simulink model "CarE_Model"  (R2019b)
settings: Solver=VariableStepAuto  StartTime=0.0  StopTime=inf  RelTol=1e-3
(part 4 of 5)

== matlab function CarE_Model/CarE_System/Emotion Module/Decay Module/Decay of Distress/MATLAB Function ==
  data: u input; y output; t input; ulast input
function y = fcn(u,t, ulast)
s = 100;
%local_t = t;

if(u == ulast)
    local_t = t-t;
else
    local_t = t-t+1;
end

if(u==0)
    y = 0;
else
    y = u -(local_t*100)/s;
end
end

== matlab function CarE_Model/CarE_System/Emotion Module/Decay Module/Decay of Fear/MATLAB Function ==
  data: u input; y output; t input; ulast input
function y = fcn(u,t, ulast)
s = 100;
%local_t = t;

if(u == ulast)
    local_t = t-t;
else
    local_t = t-t+1;
end

if(u==0)
    y = 0;
else
    y = u -(local_t*100)/s;
end
end

== matlab function CarE_Model/CarE_System/Mood Module/MATLAB Function1 ==
  data: previous_mood input; joy input; mood output; distress input; hope input; fear input; satisfaction input; fear_confirmed input; relief input; disappointment input; happy_for input; sorry_for input; gloating input; resentment input; pride input; shame input; admiration input; reproach input; gratitude input; anger input; gratification input; remorse input; liking input; disliking input; p output; n output; sort_positive output; index_positive output; sort_negative output; index_negative output; contribution output; index output; sum_of_contribution output; joy_driver input; distress_driver input; hope_driver input; fear_driver input; satisfaction_driver input; fear_confirmed_driver input; relief_driver input; disappointment_driver input; happy_for_driver input; sorry_for_driver input; gloating_driver input; resentment_driver input; pride_driver input; shame_driver input; admiration_driver input; reproach_driver input; gratitude_driver input; anger_driver input; gratification_driver input; remorse_driver input; liking_driver input; disliking_driver input
function [mood, p, n, sort_positive, index_positive, sort_negative, index_negative, contribution, index, sum_of_contribution] = mood_cal(previous_mood, joy, distress, hope, fear, satisfaction, fear_confirmed, relief, disappointment, happy_for, sorry_for, gloating, resentment, pride, shame, admiration, reproach, gratitude, anger, gratification, remorse, liking, disliking, joy_driver, distress_driver, hope_driver, fear_driver, satisfaction_driver, fear_confirmed_driver, relief_driver, disappointment_driver, happy_for_driver, sorry_for_driver, gloating_driver, resentment_driver, pride_driver, shame_driver, admiration_driver, reproach_driver, gratitude_driver, anger_driver, gratification_driver, remorse_driver, liking_driver, disliking_driver)
%psort = zeros(22,1);
positive_emo = 0;
negative_emo = 0;
individual_contribution_p = zeros(22,1);
individual_contribution_n = zeros(22,1);
positive_emo = positive_emo + abs(joy) + abs(hope) + abs(satisfaction) + abs(relief) + abs(happy_for) + abs(gloating) + abs(pride) + abs(admiration) + abs(gratitude) + abs(gratification) + abs(liking);
negative_emo = negative_emo + abs(distress) + abs(fear) + abs(fear_confirmed) + abs(disappointment) + abs(sorry_for) + abs(resentment) + abs(shame) + abs(reproach) + abs(anger) + abs(remorse) + abs(disliking);
p = positive_emo;
n = negative_emo;
if(negative_emo==0)
    negative_emo=1;
end
%% Finding the percentage contribution of each emotion in mood value
%assigning contributions to their respective arrays
%depending on if they are positive or negative
individual_contribution_p(1) = abs(joy)/positive_emo;
individual_contribution_n(2) = abs(distress)/negative_emo;
individual_contribution_p(3) = abs(hope)/positive_emo;
individual_contribution_n(4) = abs(fear)/negative_emo;
individual_contribution_p(5) = abs(satisfaction)/positive_emo;
individual_contribution_n(6) = abs(fear_confirmed)/negative_emo;
individual_contribution_p(7) = abs(relief)/positive_emo;
individual_contribution_n(8) = abs(disappointment)/negative_emo;
individual_contribution_p(9) = abs(happy_for)/positive_emo;
individual_contribution_n(10) = abs(sorry_for)/negative_emo;
individual_contribution_p(11) = abs(gloating)/positive_emo;
individual_contribution_n(12) = abs(resentment)/negative_emo;
individual_contribution_p(13) = abs(pride)/positive_emo;
individual_contribution_n(14) = abs(shame)/negative_emo;
individual_contribution_p(15) = abs(admiration)/positive_emo;
individual_contribution_n(16) = abs(reproach)/negative_emo;
individual_contribution_p(17) = abs(gratitude)/positive_emo;
individual_contribution_n(18) = abs(anger)/negative_emo;
individual_contribution_p(19) = abs(gratification)/positive_emo;
individual_contribution_n(20) = abs(remorse)/negative_emo;
individual_contribution_p(21) = abs(liking)/positive_emo;
individual_contribution_n(22) = abs(disliking)/negative_emo;

%First add the two arrays to combine the results in one array
combined_result = individual_contribution_p + individual_contribution_n;
%Sorting them in decreasing order
[contribution,index] = sort(combined_result, 'descend');
[sort_positive,index_positive] = sort(individual_contribution_p, 'descend');
[sort_negative,index_negative] = sort(individual_contribution_n, 'descend');
sum_of_contribution = sum(contribution);

%% calculating mood
if(negative_emo ~=0)
    mood = positive_emo/negative_emo;
else
    mood = previous_mood;
end

end

== matlab function CarE_Model/CarE_System/Emotion Module/Decay Module/Decay of Fear Confirmed/MATLAB Function ==
  data: u input; y output; t input; ulast input
function y = fcn(u,t, ulast)
s = 100;
%local_t = t;

if(u == ulast)
    local_t = t-t;
else
    local_t = t-t+1;
end

if(u==0)
    y = 0;
else
    y = u -(local_t*100)/s;
end
end

== matlab function CarE_Model/CarE_System/Emotion Module/Decay Module/Decay of Hope/MATLAB Function ==
  data: u input; y output; t input; ulast input
function y = fcn(u,t, ulast)
s = 100;
%local_t = t;

if(u == ulast)
    local_t = t-t;
else
    local_t = t-t+1;
end

if(u==0)
    y = 0;
else
    y = u -(local_t*100)/s;
end
end

== matlab function CarE_Model/CarE_System/Emotion Module/Decay Module/Decay of Disappointment/MATLAB Function ==
  data: u input; y output; t input; ulast input
function y = fcn(u,t, ulast)
s = 100;
%local_t = t;

if(u == ulast)
    local_t = t-t;
else
    local_t = t-t+1;
end

if(u==0)
    y = 0;
else
    y = u -(local_t*100)/s;
end
end

== matlab function CarE_Model/CarE_System/Emotion Module/Decay Module/Decay of Happy For/MATLAB Function ==
  data: u input; y output; t input; ulast input
function y = fcn(u,t, ulast)
s = 100;
%local_t = t;

if(u == ulast)
    local_t = t-t;
else
    local_t = t-t+1;
end

if(u==0)
    y = 0;
else
    y = u -(local_t*100)/s;
end
end

== matlab function CarE_Model/CarE_System/Emotion Module/Decay Module/Decay of Relief/MATLAB Function ==
  data: u input; y output; t input; ulast input
function y = fcn(u,t, ulast)
s = 100;
%local_t = t;

if(u == ulast)
    local_t = t-t;
else
    local_t = t-t+1;
end

if(u==0)
    y = 0;
else
    y = u -(local_t*100)/s;
end
end

== matlab function CarE_Model/CarE_System/Emotion Module/Decay Module/Decay of Gloating/MATLAB Function ==
  data: u input; y output; t input; ulast input
function y = fcn(u,t, ulast)
s = 100;
%local_t = t;

if(u == ulast)
    local_t = t-t;
else
    local_t = t-t+1;
end

if(u==0)
    y = 0;
else
    y = u -(local_t*100)/s;
end
end

== matlab function CarE_Model/CarE_System/Emotion Module/Decay Module/Decay of Resentment/MATLAB Function ==
  data: u input; y output; t input; ulast input
function y = fcn(u,t, ulast)
s = 100;
%local_t = t;

if(u == ulast)
    local_t = t-t;
else
    local_t = t-t+1;
end

if(u==0)
    y = 0;
else
    y = u -(local_t*100)/s;
end
end

== matlab function CarE_Model/CarE_System/Emotion Module/Decay Module/Decay of Pride/MATLAB Function ==
  data: u input; y output; t input; ulast input
function y = fcn(u,t, ulast)
s = 100;
%local_t = t;

if(u == ulast)
    local_t = t-t;
else
    local_t = t-t+1;
end

if(u==0)
    y = 0;
else
    y = u -(local_t*100)/s;
end
end

== matlab function CarE_Model/CarE_System/Emotion Module/Decay Module/Decay of Satisfaction/MATLAB Function ==
  data: u input; y output; t input; ulast input
function y = fcn(u,t, ulast)
s = 100;
%local_t = t;

if(u == ulast)
    local_t = t-t;
else
    local_t = t-t+1;
end

if(u==0)
    y = 0;
else
    y = u -(local_t*100)/s;
end
end

== matlab function CarE_Model/CarE_System/Emotion Module/Decay Module/Decay of Reproach/MATLAB Function ==
  data: u input; y output; t input; ulast input
function y = fcn(u,t, ulast)
s = 100;
%local_t = t;

if(u == ulast)
    local_t = t-t;
else
    local_t = t-t+1;
end

if(u==0)
    y = 0;
else
    y = u -(local_t*100)/s;
end
end

== matlab function CarE_Model/CarE_System/Emotion Module/Decay Module/Decay of Admiration/MATLAB Function ==
  data: u input; y output; t input; ulast input
function y = fcn(u,t, ulast)
s = 100;
%local_t = t;

if(u == ulast)
    local_t = t-t;
else
    local_t = t-t+1;
end

if(u==0)
    y = 0;
else
    y = u -(local_t*100)/s;
end
end

== matlab function CarE_Model/CarE_System/Emotion Module/Decay Module/Decay of Gratitude/MATLAB Function ==
  data: u input; y output; t input; ulast input
function y = fcn(u,t, ulast)
s = 100;
%local_t = t;

if(u == ulast)
    local_t = t-t;
else
    local_t = t-t+1;
end

if(u==0)
    y = 0;
else
    y = u -(local_t*100)/s;
end
end

== matlab function CarE_Model/CarE_System/Emotion Module/Decay Module/Decay of Anger/MATLAB Function ==
  data: u input; y output; t input; ulast input
function y = fcn(u,t, ulast)
s = 100;
%local_t = t;

if(u == ulast)
    local_t = t-t;
else
    local_t = t-t+1;
end

if(u==0)
    y = 0;
else
    y = u -(local_t*100)/s;
end
end

== matlab function CarE_Model/CarE_System/Emotion Module/Decay Module/Decay of Gratification/MATLAB Function ==
  data: u input; y output; t input; ulast input
function y = fcn(u,t, ulast)
s = 100;
%local_t = t;

if(u == ulast)
    local_t = t-t;
else
    local_t = t-t+1;
end

if(u==0)
    y = 0;
else
    y = u -(local_t*100)/s;
end
end

== matlab function CarE_Model/CarE_System/Emotion Module/Decay Module/Decay of Remorse/MATLAB Function ==
  data: u input; y output; t input; ulast input
function y = fcn(u,t, ulast)
s = 100;
%local_t = t;

if(u == ulast)
    local_t = t-t;
else
    local_t = t-t+1;
end

if(u==0)
    y = 0;
else
    y = u -(local_t*100)/s;
end
end

== matlab function CarE_Model/CarE_System/Emotion Module/Decay Module/Decay of Liking/MATLAB Function ==
  data: u input; y output; t input; ulast input
function y = fcn(u,t, ulast)
s = 100;
%local_t = t;

if(u == ulast)
    local_t = t-t;
else
    local_t = t-t+1;
end

if(u==0)
    y = 0;
else
    y = u -(local_t*100)/s;
end
end

== matlab function CarE_Model/CarE_System/Emotion Module/Decay Module/Decay of Disliking/MATLAB Function ==
  data: u input; y output; t input; ulast input
function y = fcn(u,t, ulast)
s = 100;
%local_t = t;

if(u == ulast)
    local_t = t-t;
else
    local_t = t-t+1;
end

if(u==0)
    y = 0;
else
    y = u -(local_t*100)/s;
end
end

== matlab function CarE_Model/CarE_System/Emotion Module/Decay Module/Decay of Shame/MATLAB Function ==
  data: u input; y output; t input; ulast input
function y = fcn(u,t, ulast)
s = 100;
%local_t = t;

if(u == ulast)
    local_t = t-t;
else
    local_t = t-t+1;
end

if(u==0)
    y = 0;
else
    y = u -(local_t*100)/s;
end
end

== matlab function CarE_Model/CarE_System/Emotion Module/Intensity Module/MATLAB Function to calculate individual emotion intensity ==
  data: goal_id input; agent_id input; event_id input; action_id input; LoS_0 input; LoF_0 input; fix input; joy output; distress output; hope output; fear output; satisfaction output; fear_confirmed output; relief output; disappointment output; happy_for output; sorry_for output; gloating output; resentment output; pride output; shame output; admiration output; reproach output; gratitude output; anger output; gratification output; remorse output; liking output; disliking output; sout output; fout output; sin input; fin input
function [joy, distress, hope, fear, satisfaction, fear_confirmed, relief, disappointment, happy_for, sorry_for, gloating, resentment, pride, shame, admiration, reproach, gratitude, anger, gratification, remorse, liking, disliking, sout, fout] = intensity_cal(goal_id, agent_id, event_id, action_id,LoS_0, LoF_0 , fix, sin, fin)
%% INITIALIZING
intensity.joy = 0;
intensity.distress = 0;
intensity.hope = 0;
intensity.fear = 0;
intensity.satisfaction = 0;
intensity.fear_confirmed = 0;
intensity.relief = 0;
intensity.disappointment = 0;
intensity.happy_for = 0;
intensity.sorry_for = 0;
intensity.gloating = 0;
intensity.resentment = 0;
intensity.pride = 0;
intensity.shame = 0;
intensity.admiration = 0;
intensity.reproach = 0;
intensity.gratitude = 0;
intensity.anger = 0;
intensity.gratification = 0;
intensity.remorse = 0;
intensity.liking = 0;
intensity.disliking = 0;

joy = 0;
distress = 0;
hope = 0;
fear = 0;
satisfaction = 0;
fear_confirmed = 0;
relief = 0;
disappointment = 0;
happy_for = 0;
sorry_for = 0;
gloating = 0;
resentment = 0;
pride = 0;
shame = 0;
admiration = 0;
reproach = 0;
gratitude = 0;
anger = 0;
gratification = 0;
remorse = 0;
liking = 0;
disliking = 0;

%% Defining LoS and LoF fix or as te stress factor
LoS=0.5;
LoF=0.5;
%fix=1;
coder.extrinsic('Cal_LoS')
[LoS,LoF]=Cal_LoS(goal_id,LoS_0, LoF_0 , fix);

%% DEFINING DATASET ARRAYS
%goal_set = [id number, name, hierarchy, desirability of success, desirability of not to fail, likelihood of success, likelihood of failure, related agent id];
goal_set = [
1, 100, 100, 100, 0.5, 0.5, 1; %"Stay under speed limit"
2, 95, 80, 70, LoS, LoF, 3;     %"Maintain proper distance with agents"
3, 85, 90, 75, LoS, LoF, 4;     %"Perform proper lane changes"
4, 100, 100, 100, 1, 0, 5;      %"Stop at red traffic light"
5, 95, 95, 90, 0.5, 0.5, 4;     %"Yield before turning"
6, 100, 100, 100, 1, 0, 6;     %"Avoid collision with pedestrians"
7, 100, 100, 100, LoS, LoF, 6;     %"Avoid collision with vehicles"
8, 85, 90, 75, LoS, LoF, 4];       % "Perform proper curve management"

%agent_set = [id number, name, type not_human|human, appealiness, related goal id];
agent_set = [1, 1, 100, -1;   %"ME (car itself)"
2, 1, 100, -1;              %"Driver"
3, 1, 90, 2;                %"Vehicle in front",
4, 1, 90, 2;                %"Vehicle in back" 
5, 0, 80, 4;                %"Traffic lights" 
6, 1, 100, 6;               %"Pedestrians" 
7, 0, 80, 6;                %"Animals" 
8, 0, 80, 6];               %"Buildings"

%event_set = [id number	name, change in goal LoS, change in goal LoF, related goal id];
event_set = [1, 1, -1, 1;   %"Staying under speed limit" 
2, -1, 1, 1;        %"Overspeeding detected" 
3, 1, -1, 2;        %"Proper distance maintained with agents" 
4, -1, 1, 2;        %"Improper distance maintained with agents"
5, 1, -1, 3;        %"Proper lane change performed" 
6, -0.75, 0.75, 3;  %"Improper lane change performed" 
7, 1, -1, 4;        %"Stopped at red light" 
8, -1, 1, 4;        %"Drove past red light" 
9, 1, -1, 5;        %"Yielded before turning" 
10, -0.5, 0.5, 5;   %"Turned without yielding" 
11, 1, -1, 6;       %"No collision detected" 
12, -1, 1, 6;      %"Collision detected" 
13, 1, -1, 3;        %"Proper curve handle performed" 
14, -0.75, 0.75, 3];  %"Improper curve handle performed" 

%action_set = [id number, name, praiseworthiness, related agent id, responsibility of the agent, related event id];
action_set = [1,  100, 2, 1, 1; %"I stayed in speed limit"
2, -90, 2, 1, 2;    %"I overspeeded" 
3, 100, 3, 1, 3;    %"I maintained proper distance with agents" 
4, -100, 3, 1, 4;    %"I maintained improper distance with agents" 
5, 80, 4, 1, 5;    %"I performed proper lane change" 
6, -80, 4, 1, 6;     %"I performed improper lane change" 
7, 100, 5, 1, 7;    %"I stopped at red light" 
8, -100, 5, 1, 8;    %"I drove past red light" 
9, 80, 4, 1, 9;   %"I yielded before turning" 
10, -80, 4, 1, 10;   %"I turned without yielding" 
11, 100, 6, 1, 11;   %"I detected no collision" 
12, -100, 6, 1, 12; %"I detected a collision" 
13, 90, 4, 1, 13;    %"I performed proper curve handle" 
14, -90, 4, 1, 14];     %"I performed improper curve handle" 

%% DEFINING STRUCTURES AND VARIABLES
%% ASSIGNING IMPORTED DATA TO VARIABLES
%GOAL
%if(goal_id ~= 0)
    goal.id = goal_set(goal_id,1);
    %goal.name = goal_set(goal_id,2);
    goal.hierarchy = goal_set(goal_id,2);
    goal.DoS = goal_set(goal_id,3);
    goal.DnF = goal_set(goal_id,4);
    goal.LoS = goal_set(goal_id,5);
    goal.LoF = goal_set(goal_id,6);
    goal.agent = goal_set(goal_id,7);
%end

%AGENT
%if(agent_id ~= 0)
    agent.id = agent_set(agent_id,1);
    %agent.name = agent_set(agent_id,2);
    agent.type = agent_set(agent_id,2);
    agent.appeal = agent_set(agent_id,3);
    agent.goal = agent_set(agent_id,4);
%end

%EVENT
%if(event_id ~= 0)
    event.id = event_set(event_id,1);
    %event.name = event_set(event_id,2);
    event.dLoS = event_set(event_id,2);
    event.dLoF = event_set(event_id,3);
    event.goal = event_set(event_id,4);
%end

%ACTION
%if(action_id ~= 0)
    action.id = action_set(action_id,1);
    %action.name = action_set(action_id,2);
    action.praise = action_set(action_id,2);
    action.agent = action_set(action_id,3);
    action.resp = action_set(action_id,4);
    action.event = action_set(action_id,5);
%end
sout = goal.LoS;
fout = goal.LoF;
last.LoS = sin;
last.LoF = fin;
% last.LoS = 0.5;
% last.LoF = 0.5;
no_emotion = 0;


%% FINDING EMOTION INTENSITY VALUES

% HOPE OR FEAR
if(goal.LoS > goal.LoF)
    intensity.hope = goal.LoS * goal.DoS;
    hope = intensity.hope;
    intensity.fear = no_emotion;
    fear = intensity.fear;
else
    intensity.fear = goal.LoF * goal.DnF;
    fear = intensity.fear;
    intensity.hope = no_emotion;
    hope = intensity.hope;
end

% LIKE OR DISLIKE
if(agent.appeal > 0)
    intensity.liking = agent.appeal;
    liking = intensity.liking;
    intensity.disliking = no_emotion;
    disliking = intensity.disliking;
else
    intensity.disliking = agent.appeal;
    disliking = intensity.disliking;
    intensity.liking = no_emotion;
    liking = intensity.liking;
end

% PRIDE OR SHAME - ADMIRATION OR REPROACH
if(agent.id==1)
    intensity.admiration = no_emotion;
    admiration = intensity.admiration;
    intensity.reproach = no_emotion;
    reproach = intensity.reproach;
    if(action.praise>0)
        intensity.pride = action.praise;
        pride = intensity.pride;
        intensity.shame = no_emotion;
        shame = intensity.shame;
    else
        intensity.shame = action.praise;
        shame = intensity.shame;
        intensity.pride = no_emotion;
        pride = intensity.pride;
    end
elseif(agent.id~=0)
    intensity.pride = no_emotion;
    pride = intensity.pride;
    intensity.shame = no_emotion;
    shame = intensity.shame;
    if(action.praise>0)
        intensity.admiration = action.praise;
        admiration = intensity.admiration;
        intensity.reproach = no_emotion;
        reproach = intensity.reproach;
    else
        intensity.reproach = action.praise;
        reproach = intensity.reproach;
        intensity.admiration = no_emotion;
        admiration = intensity.admiration;
    end
end

% GRATIFICATION OR GRATITUDE - REMORSE OR ANGER
if(event.dLoS > 0 && event.dLoF <= 0)
    intensity.remorse = no_emotion;
    remorse = intensity.remorse;
    intensity.anger = no_emotion;
    anger = intensity.anger;
	if(agent.id == 1)
		intensity.gratification = goal.DoS * action.resp;
    	gratification = intensity.gratification;
		intensity.gratitude = no_emotion;
    	gratitude = intensity.gratitude;
	else
		intensity.gratitude = goal.DoS * action.resp;
    	gratitude = intensity.gratitude;
		intensity.gratification = no_emotion;
   		gratification = intensity.gratification;
	end
else
    intensity.gratification = no_emotion;
   	gratification = intensity.gratification;
    intensity.gratitude = no_emotion;
    gratitude = intensity.gratitude;
    if(event.dLoF > 0 && event.dLoS <= 0)
        if(agent.id == 1)
            intensity.remorse = goal.DnF * action.resp;
            remorse = intensity.remorse;
            intensity.anger = no_emotion;
            anger = intensity.anger;
        else
            intensity.anger = goal.DnF * action.resp;
            anger = intensity.anger;
            intensity.remorse = no_emotion;
            remorse = intensity.remorse;
        end
    else
        intensity.gratification = no_emotion;
        gratification = intensity.gratification;
        intensity.gratitude = no_emotion;
        gratitude = intensity.gratitude;        
        intensity.remorse = no_emotion;
        remorse = intensity.remorse;
        intensity.anger = no_emotion;
        anger = intensity.anger;

    end
end

%JOY OR DISTRESS - HAPPY-FOR OR RESENTMENT - SORRY-FOR OR GLOATING
if(agent.id == 1)
    intensity.happy_for = no_emotion;
    happy_for = intensity.happy_for;
    intensity.resentment = no_emotion;
    resentment = intensity.resentment;
    intensity.sorry_for = no_emotion;
    sorry_for = intensity.sorry_for;
    intensity.gloating = no_emotion;
    gloating = intensity.gloating;
    if(event.dLoS>0 && event.dLoF<=0)
        intensity.joy = event.dLoS * goal.DoS;
        joy = intensity.joy;
        intensity.distress = no_emotion;
        distress = intensity.distress;
    else
        intensity.joy = no_emotion;
        joy = intensity.joy;
        if(event.dLoF>0 && event.dLoS<=0)
            intensity.distress = event.dLoF * goal.DnF;
            distress = intensity.distress;
        else
            intensity.joy = no_emotion;
            joy = intensity.joy;
            intensity.distress = no_emotion;
            distress = intensity.distress;
        end
    end
elseif(agent.id~=1)
    intensity.joy = no_emotion;
    joy = intensity.joy;
    intensity.distress = no_emotion;
    distress = intensity.distress;
    if(event.dLoS>0 && event.dLoF<=0)
        intensity.sorry_for = no_emotion;
        sorry_for = intensity.sorry_for;
        intensity.gloating = no_emotion;
        gloating = intensity.gloating;
        if(agent.appeal>0)
            intensity.happy_for = abs(agent.appeal) * event.dLoS * goal.DoS;
            happy_for = intensity.happy_for;
            intensity.resentment = no_emotion;
            resentment = intensity.resentment;
        else
            intensity.resentment = abs(agent.appeal) * event.dLoS * goal.DoS;
            resentment = intensity.resentment;
            intensity.happy_for = no_emotion;
            happy_for = intensity.happy_for;
        end
    else
        intensity.happy_for = no_emotion;
        happy_for = intensity.happy_for;
        intensity.resentment = no_emotion;
        resentment = intensity.resentment;
        if(event.dLoF>0 && event.dLoS<=0)
            if(agent.appeal>0)
                intensity.sorry_for = abs(agent.appeal) * event.dLoF * goal.DnF;
                sorry_for = intensity.sorry_for;
                intensity.gloating = no_emotion;
                gloating = intensity.gloating;
            else
                intensity.gloating = abs(agent.appeal) * event.dLoF * goal.DnF;
                gloating = intensity.gloating;
                intensity.sorry_for = no_emotion;
                sorry_for = intensity.sorry_for;
            end
        else
            intensity.happy_for = no_emotion;
            happy_for = intensity.happy_for;
            intensity.resentment = no_emotion;
            resentment = intensity.resentment;
            intensity.sorry_for = no_emotion;
            sorry_for = intensity.sorry_for;
            intensity.gloating = no_emotion;
            gloating = intensity.gloating;
        end
    end
end

%SATISFACTION OR DISAPPOINTMENT - FEAR-CONFIRMED OR RELIEF
if(last.LoS > last.LoF)
    intensity.fear_confirmed = no_emotion;
    fear_confirmed = intensity.fear_confirmed;
    intensity.relief = no_emotion;
    relief = intensity.relief;
    if(goal.LoS == 1)
        intensity.satisfaction = last.LoS * goal.DoS;
        satisfaction = intensity.satisfaction;
        intensity.disappointment = no_emotion;
        disappointment = intensity.disappointment;
    else
        intensity.satisfaction = no_emotion;
        satisfaction = intensity.satisfaction;
        if(goal.LoF == 1)
            intensity.disappointment = last.LoS * goal.DoS;
            disappointment = intensity.disappointment;
        else
            intensity.satisfaction = no_emotion;
            satisfaction = intensity.satisfaction;
            intensity.disappointment = no_emotion;
            disappointment = intensity.disappointment;
        end
    end
else
    intensity.satisfaction = no_emotion;
    satisfaction = intensity.satisfaction;
    intensity.disappointment = no_emotion;
    disappointment = intensity.disappointment;
    if(goal.LoS == 1)
        intensity.relief = last.LoF * goal.DnF;
        relief = intensity.relief;
        intensity.fear_confirmed = no_emotion;
        fear_confirmed = intensity.fear_confirmed;
    else
        intensity.relief = no_emotion;
        relief = intensity.relief;
        if(goal.LoF == 1)
            intensity.fear_confirmed = last.LoF * goal.DnF;
            fear_confirmed = intensity.fear_confirmed;
        else
            intensity.relief = no_emotion;
            relief = intensity.relief;
            intensity.fear_confirmed = no_emotion;
            fear_confirmed = intensity.fear_confirmed;
        end
    end
end

%% NORMALIZED VALUES
joy = inter(joy, 0, 100);
distress = inter(distress, 0, 100);
hope = inter(hope, 0, 100);
fear = inter(fear, 0, 100);
satisfaction = inter(satisfaction, 0, 100);
fear_confirmed = inter(fear_confirmed, 0, 100);
relief = inter(relief, 0, 100);
disappointment = inter(disappointment, 0, 100);
happy_for = inter(happy_for, 0, 10000);     %these values were too big and had to be interpolated to fit in 0-100 range
sorry_for = inter(sorry_for, 0, 10000);
gloating = inter(gloating, 0, 10000);
resentment = inter(resentment, 0, 10000);
pride = inter(pride, 0, 100);
shame = inter(shame, 0, 100);
admiration = inter(admiration, 0, 100);
reproach = inter(reproach, 0, 100);
gratitude = inter(gratitude, 0, 100);
anger = inter(anger, 0, 100);
gratification = inter(gratification, 0, 100);
remorse = inter(remorse, 0, 100);
liking = inter(liking, 0, 100);
disliking = inter(disliking, 0, 100);

%% NORMALIZING VALUES
% INTERPOLATION FUNCTION NEW
function interpolated = inter(a_val, low_th, high_th)
    if(a_val<0)
        y1 = -100;
        %y2 = 0;
        y3 = 0;
        x1 = -high_th;
        x2 = a_val;
        x3 = -low_th;
    else
        y1 = 100;
        %y2 = 0;
        y3 = 0;
        x1 = high_th;
        x2 = a_val;
        x3 = low_th;
    end
    %calculate the interpolated value    
    y2 = (((x2-x1)*(y3-y1))/(x3-x1))+y1;
    interpolated = y2;
end

end

== matlab function CarE_Model/CarE_System/Emotion Module/Decay Module/Decay of Joy/MATLAB Function1 ==
  data: u input; y output; t input; ulast input
function y = fcn(u,t, ulast)
% u - emotion intensity value
% ulast - emotion intensity in last instance of time
% t - timer value (age of emotion)
% s - max decay time
% y - decayed emotion intensity
s = 100;

if(u == ulast)
    local_t = t-t;
else
    local_t = t-t+1;
end

if(u==0)
    y = 0;
else
    y = u -(local_t*100)/s;
end
end

== matlab function CarE_Model/CarE_System/Emotion Module/Decay Module/Decay of Sorry For/MATLAB Function ==
  data: u input; y output; t input; ulast input
function y = fcn(u,t, ulast)
s = 100;
%local_t = t;

if(u == ulast)
    local_t = t-t;
else
    local_t = t-t+1;
end

if(u==0)
    y = 0;
else
    y = u -(local_t*100)/s;
end
end

== matlab function CarE_Model/CarE_System/Input_module_2.0/MATLAB Function ==
  data: distance input; brakes_st output; serv_brake_PE_st output; second_brake_st output; parking_brake_st output; axle_st output; warn_lamp_st output; door_st output; fog_lamp_st output; headlamp_st output; reverse_lamp_st output; belts_st output; airbag_st output; seat_st output; steering_st output; wheel_alignment_st output; EPS_st output; Steering_wheel_st output; stop_lamp_st output; suspension_st output; Telltales_st output; wheel_hub_st output; wheel_st output; tyre_st output; cabine_st output; chassis_st output
function [brakes_st,serv_brake_PE_st,second_brake_st,parking_brake_st,axle_st,warn_lamp_st,door_st,fog_lamp_st,headlamp_st,reverse_lamp_st,belts_st,airbag_st,seat_st,steering_st,wheel_alignment_st,EPS_st,Steering_wheel_st,stop_lamp_st,suspension_st,Telltales_st,wheel_hub_st,wheel_st,tyre_st,cabine_st,chassis_st]= state_VH(distance)
coder.extrinsic('VH_fun_state')
brakes_st=1;
serv_brake_PE_st=1;
second_brake_st=1;
parking_brake_st=1;
axle_st=1;
warn_lamp_st=1;
door_st=1;
fog_lamp_st=1;
headlamp_st=1;
reverse_lamp_st=1;
belts_st=1;
airbag_st=1;
seat_st=1;
steering_st=1;
wheel_alignment_st=1;
EPS_st=1;
Steering_wheel_st=1;
stop_lamp_st=1;
suspension_st=1;
Telltales_st=1;
wheel_hub_st=1;
wheel_st=1;
tyre_st=1;
cabine_st=1;
chassis_st=1;

[brakes_st,serv_brake_PE_st,second_brake_st,parking_brake_st,axle_st,warn_lamp_st,door_st,fog_lamp_st,headlamp_st,reverse_lamp_st,belts_st,airbag_st,seat_st,steering_st,wheel_alignment_st,EPS_st,Steering_wheel_st,stop_lamp_st,suspension_st,Telltales_st,wheel_hub_st,wheel_st,tyre_st,cabine_st,chassis_st]= VH_fun_state(distance);
end

== matlab function CarE_Model/CarE_System/Input_module_2.0/MATLAB Function1 ==
  data: avg_gap input; gap_st output; gap input
function gap_st  = gap_st_fun(avg_gap,gap)
coder.extrinsic('gap_st_comp');
gap_st=1;
gap_st  = gap_st_comp(avg_gap,gap);

end

== matlab function CarE_Model/CarE_System/Input_module_2.0/MATLAB Function2 ==
  data: obt_recog input; ob_recog_st output
function ob_recog_st = ob_recog_st_fun(obt_recog)
    coder.extrinsic('ob_recog_st_comp');
    ob_recog_st=1;
       ob_recog_st = ob_recog_st_comp(obt_recog);
end

== matlab function CarE_Model/CarE_System/Input_module_2.0/MATLAB Function3 ==
  data: acc_road_today input; prob_acc_road_st output; mean_acc input; SD_acc_road input
function prob_acc_road_st = prob_acc_road_st_funtion(acc_road_today,mean_acc,SD_acc_road)
    
    coder.extrinsic('prob_acc_road_st_fun');
      %coder.extrinsic('normcdf');
      prob_acc_road_st=1;
    prob_acc_road_st = prob_acc_road_st_fun(acc_road_today,mean_acc,SD_acc_road);
end

== matlab function CarE_Model/CarE_System/Health_Module_2.0/MATLAB Function ==
  data: driver_age_st input; HealthFactor output; driver_alcohol_st input; driver_alertness_st input; driver_vision_st input; driver_work_load_st input; driver_emotion_st input; driver_attitude_st input; maintenance_periodicity_st input; gap_st input; speeding_freq_st input; vehicle_mass_st input; brakes_st input; serv_brake_PE_st input; second_brake_st input; parking_brake_st input; axle_st input; warn_lamp_st input; door_st input; fog_lamp_st input; headlamp_st input; reverse_lamp_st input; belts_st input; airbag_st input; seat_st input; steering_st input; wheel_alignment_st input; EPS_st input; Steering_wheel_st input; stop_lamp_st input; suspension_st input; Telltales_st input; wheel_hub_st input; wheel_st input; tyre_st input; cabine_st input; chassis_st input; noise_st input; obt_recog_st input; v2v_st input; v2i_st input; friendly_HM_interaction_st input; software_freq_st input; biddata_connection_st input; digital_user_interface_st input; cooperative_driving_st input; road_surface_st input; road_condition_st input; prob_acc_road_st input; prob_contruction_st input; cab_temperature_st input; cab_humidity_st input; driving_env_condition_st input; weather_st input; time_of_day_st input; check_if_hit input; check_collision input
function HealthFactor = HeatlFactor_fun(driver_age_st,driver_alcohol_st,driver_alertness_st,driver_vision_st,driver_work_load_st,driver_emotion_st,driver_attitude_st,maintenance_periodicity_st,gap_st,speeding_freq_st,vehicle_mass_st,brakes_st,serv_brake_PE_st,second_brake_st,parking_brake_st,axle_st,warn_lamp_st,door_st,fog_lamp_st,headlamp_st,reverse_lamp_st,belts_st,airbag_st,seat_st,steering_st,wheel_alignment_st,EPS_st,Steering_wheel_st,stop_lamp_st,suspension_st,Telltales_st,wheel_hub_st,wheel_st,tyre_st,cabine_st,chassis_st,noise_st,obt_recog_st,v2v_st,v2i_st,friendly_HM_interaction_st,software_freq_st,biddata_connection_st,digital_user_interface_st,cooperative_driving_st,road_surface_st,road_condition_st,prob_acc_road_st,prob_contruction_st,cab_temperature_st,cab_humidity_st,driving_env_condition_st,weather_st,time_of_day_st,check_if_hit,check_collision)
HealthFactor=1;
coder.extrinsic('HealthFactor_fn')

HealthFactor = HealthFactor_fn(driver_age_st,driver_alcohol_st,driver_alertness_st,driver_vision_st,driver_work_load_st,driver_emotion_st,driver_attitude_st,maintenance_periodicity_st,gap_st,speeding_freq_st,vehicle_mass_st,brakes_st,serv_brake_PE_st,second_brake_st,parking_brake_st,axle_st,warn_lamp_st,door_st,fog_lamp_st,headlamp_st,reverse_lamp_st,belts_st,airbag_st,seat_st,steering_st,wheel_alignment_st,EPS_st,Steering_wheel_st,stop_lamp_st,suspension_st,Telltales_st,wheel_hub_st,wheel_st,tyre_st,cabine_st,chassis_st,noise_st,obt_recog_st,v2v_st,v2i_st,friendly_HM_interaction_st,software_freq_st,biddata_connection_st,digital_user_interface_st,cooperative_driving_st,road_surface_st,road_condition_st,prob_acc_road_st,prob_contruction_st,cab_temperature_st,cab_humidity_st,driving_env_condition_st,weather_st,time_of_day_st,check_if_hit,check_collision);


end

== matlab function CarE_Model/CarE_System/Event_detect_module/MATLAB Function ==
  data: egocar_x input; event_id output; egocar_z input; egocar_rot input; olanecar_presence input; leadcar_presence input; turn_trigger input
function event_id = Event_recognition(egocar_x,egocar_z,egocar_rot,olanecar_presence, leadcar_presence,turn_trigger)

%straight line lane change
%ode_wide=8; %unity units
event_id=1;
coder.extrinsic('Event_identification');
event_id = Event_identification(egocar_x,egocar_z,egocar_rot,olanecar_presence, leadcar_presence,turn_trigger);

%{
w_ego_car=1.58; %unity units
lanechange_trigger=0;
    if egocar_rot>=45 && egocar_rot<=135      
        lane_position=816;%z coordinate
        egocar_l=egocar_z-w_ego_car/2;
        egocar_r=egocar_z+w_ego_car/2; 
        direction=1;
    elseif egocar_rot>=225 && egocar_rot<=315
        lane_position=962; %z coordianates
        egocar_l=egocar_z+w_ego_car/2;
        egocar_r=egocar_z-w_ego_car/2;
        direction=-1;
    elseif egocar_rot>135 && egocar_rot<225
        lane_position=954;%xcoordinates
        egocar_l=egocar_x-w_ego_car/2;
        egocar_r=egocar_x+w_ego_car/2;
        direction=1;
    elseif egocar_rot>315 && egocar_rot<=360 || egocar_rot>=0 && egocar_rot<45
        lane_position=752.5;%xcoordinates
         egocar_l=egocar_x+w_ego_car/2;
        egocar_r=egocar_x-w_ego_car/2;
        direction=-1;
    end
    
     if egocar_l>lane_position && direction==1 || egocar_r<lane_position && direction==1
           lanechange_trigger=0;
     elseif egocar_l<lane_position && direction==-1 || egocar_r>lane_position && direction==-1
           lanechange_trigger=0;
     end
      
     if  direction ==1 && egocar_l<=lane_position && egocar_r>=lane_position
         lanechange_trigger=1;
     elseif direction ==-1 && egocar_l>=lane_position && egocar_r<=lane_position
         lanechange_trigger=1;
     end


    if olanecar_presence==1 && leadcar_presence==1 && lanechange_trigger==1 || olanecar_presence==0 && leadcar_presence==1 && lanechange_trigger==1
            event_id=5;
    elseif olanecar_presence==0 && leadcar_presence==1 && lanechange_trigger==0
            event_id=4;
    elseif lanechange_trigger==1 && olanecar_presence==0 && leadcar_presence==0 && turn_trigger==0
            event_id=3;
    elseif turn_trigger==1 && olanecar_presence==0 && leadcar_presence==0
            event_id=2;
    else
        event_id=1;
    end
    %}
end

== matlab function CarE_Model/CarE_System/Personality_module/MATLAB Function ==
  data: speed input; x output; max_speed input; max_x output
function [x,max_x] = Gain_fun(speed,max_speed)

    x=speed;
    max_x=max_speed;
end

== matlab function CarE_Model/CarE_System/Personality_module/MATLAB Function1 ==
  data: x input; U output; r input; max_x input
function U = Utility_fun(x,r,max_x)

    if x==0
        U_temp=0;
    else
        if r>=1
            r=0.999;
        end
        U_temp=((x)^(1-r))/(1-r);
    end
        max_U=((max_x)^(1-r))/(1-r);
        U=U_temp/max_U;

end

== matlab function CarE_Model/CarE_System/Stress_module/MATLAB Function ==
  data: distance input; SF_VH output
function SF_VH  = SF_VH_fun(distance)
    SF_VH=0;
    coder.extrinsic('SfactorVH_fun')
    SF_VH=SfactorVH_fun(distance);

end

== matlab function CarE_Model/CarE_System/Stress_module/MATLAB Function1 ==
  data: Mean_acc_road input; SF_Env output; SD_acc_road input; acc_road_today input; road_surface_st input; road_cond_st input; weather_st input; time_day_st input; egocar_speed input; avgspeed_data input
function SF_Env = SF_Env_fun(Mean_acc_road,SD_acc_road,acc_road_today,road_surface_st,road_cond_st,weather_st,time_day_st,egocar_speed,avgspeed_data)
    SF_Env=0;
    coder.extrinsic('SfactorEnv_fun')
    SF_Env=SfactorEnv_fun(Mean_acc_road,SD_acc_road,acc_road_today,road_surface_st,road_cond_st,weather_st,time_day_st,egocar_speed,avgspeed_data);
end

== matlab function CarE_Model/CarE_System/Stress_module/MATLAB Function2 ==
  data: Prob_obj_detec input; SF_VC output; v2v_st input; v2i_st input; bd_conect_st input; coop_auto_st input
function SF_VC  = SF_VC_fun(Prob_obj_detec,v2v_st,v2i_st,bd_conect_st,coop_auto_st)
    SF_VC=0;
    coder.extrinsic('SfactorVC_fun')
    SF_VC=SfactorVC_fun(Prob_obj_detec,v2v_st,v2i_st,bd_conect_st,coop_auto_st);
end

== matlab function CarE_Model/CarE_System/Stress_module/MATLAB Function3 ==
  data: speed_ecar input; SF_driving output; a_vehicle input; event_id input; gravity input; avg_speed input; rate_acc input; rate_desacc input; crit_gap input; pos_ecar_x input; pos_ecar_z input; rot_ecar input; pos_lead_car_x input; pos_lead_car_z input; speed_lead_car input; olanecar_presence input; pos_olane_car_x input; pos_olane_car_z input; rot_olane_car input; speed_olane_car input; gap output; check_if_hit input; collisiondetection input
function  [SF_driving,gap]= SF_driving_fun(speed_ecar,a_vehicle,event_id,gravity,avg_speed,rate_acc,rate_desacc,crit_gap,pos_ecar_x,pos_ecar_z,rot_ecar,pos_lead_car_x,pos_lead_car_z,speed_lead_car,olanecar_presence,pos_olane_car_x,pos_olane_car_z,rot_olane_car,speed_olane_car,check_if_hit,collisiondetection)
%%%%%%%%%%%%%%%%%%%%%%%%%%%%%%%%%%%%%
%{
possible events:
- driving alone
    -straingt line. event_id=1
    -curve. event_id=2
    -lane change. event_id=3 
- driving with another car
    -following another car. event_id=4
    -overtake. event_id=5
%}
%%%%%%%%%%%%%%%%%%%%%%%%%%%%%%%%%%%%%
    SF_driving=0;
    gap=1;
    coder.extrinsic('SF_driving_fun') 
    [SF_driving,gap]= SF_driving_fun(speed_ecar,a_vehicle,event_id,gravity,avg_speed,rate_acc,rate_desacc,crit_gap,pos_ecar_x,pos_ecar_z,rot_ecar,pos_lead_car_x,pos_lead_car_z,speed_lead_car,olanecar_presence,pos_olane_car_x,pos_olane_car_z,rot_olane_car,speed_olane_car,check_if_hit,collisiondetection);
end

== matlab function CarE_Model/CarE_System/Stress_module/MATLAB Function4 ==
  data: SF_VH input; SF output; SF_Env input; SF_VC input; SF_driving input
function SF = SF_cal(SF_VH,SF_Env,SF_VC,SF_driving)
    P1=SF_VH+SF_Env-SF_VH*SF_Env;
    P2=P1+SF_VC-P1*SF_VC;
    %SF=SF_VC+SF_Env+SF_VH+SF_driving-(SF_VC*SF_Env+SF_VC*SF_VH+SF_VH*SF_Env+SF_driving*SF_VC+SF_driving*SF_Env+SF_driving*SF_VH)+SF_VH*SF_Env*SF_VC*SF_driving;
    SF=P2+SF_driving-P2*SF_driving;
end

== matlab function CarE_Model/CarE_System/Emotion_Intensity_Input_Module/MATLAB Function ==
  data: event_0 input; goal_id output; event_detected input; sf_total input; check_hit input; check_trigger input; check_collision input; gap_st input; egocar_speed input; agent_id output; event_id output; action_id output; LoS output; LoF output; max_speed input
function [goal_id,agent_id,event_id,action_id,LoS,LoF] = Intensity_input(event_0,event_detected,sf_total,  check_hit,check_trigger,check_collision,gap_st,egocar_speed,max_speed)
  
  goal_id=1;
  agent_id=1;
  event_id=1;
  action_id=1;
  LoS=0.5;
  LoF=0.5;
  coder.extrinsic('e_intensity_detect');
[goal_id,agent_id,event_id,action_id,LoS,LoF] = e_intensity_detect(event_0,event_detected,sf_total,check_hit,check_trigger,check_collision,gap_st,egocar_speed,max_speed);
        
     



    end

== matlab function CarE_Model/CarE_System/Input_module_2.0/MATLAB Function4 ==
  data: driver_age_st input; driver_alcohol_st input; driver_alertness_st input; driver_vision_st input; driver_work_load_st input; driver_emotion_st input; driver_attitude_st input; maintenance_periodicity_st input; gap_st input; speeding_freq_st input; vehicle_mass_st input; brakes_st input; serv_brake_PE_st input; second_brake_st input; parking_brake_st input; axle_st input; warn_lamp_st input; door_st input; fog_lamp_st input; headlamp_st input; reverse_lamp_st input; belts_st input; airbag_st input; seat_st input; steering_st input; wheel_alignment_st input; EPS_st input; Steering_wheel_st input; stop_lamp_st input; suspension_st input; Telltales_st input; wheel_hub_st input; wheel_st input; tyre_st input; cabine_st input; chassis_st input; noise_st input; obt_recog_st input; v2v_st input; v2i_st input; friendly_HM_interaction_st input; software_freq_st input; biddata_connection_st input; digital_user_interface_st input; cooperative_driving_st input; road_surface_st input; road_condition_st input; prob_acc_road_st input; prob_contruction_st input; cab_temperature_st input; cab_humidity_st input; driving_env_condition_st input; weather_st input; time_of_day_st input; driver_age_st output; check_if_hit input; check_collision input; driver_alcohol_st output; driver_alertness_st output; driver_vision_st output; driver_work_load_st output; driver_emotion_st output; driver_attitude_st output; maintenance_periodicity_st output; gap_st output; speeding_freq_st output; vehicle_mass_st output; brakes_st output; serv_brake_PE_st output; second_brake_st output; parking_brake_st output; axle_st output; warn_lamp_st output; door_st output; fog_lamp_st output; headlamp_st output; reverse_lamp_st output; belts_st output; airbag_st output; seat_st output; steering_st output; wheel_alignment_st output; EPS_st output; Steering_wheel_st output; stop_lamp_st output; suspension_st output; Telltales_st output; wheel_hub_st output; wheel_st output; tyre_st output; cabine_st output; chassis_st output; noise_st output; obt_recog_st output; v2v_st output; v2i_st output; friendly_HM_interaction_st output; software_freq_st output; biddata_connection_st output; digital_user_interface_st output; cooperative_driving_st output; road_surface_st output; road_condition_st output; prob_acc_road_st output; prob_contruction_st output; cab_temperature_st output; cab_humidity_st output; driving_env_condition_st output; weather_st output; time_of_day_st output
function [driver_age_st,driver_alcohol_st,driver_alertness_st,driver_vision_st,driver_work_load_st,driver_emotion_st,driver_attitude_st,maintenance_periodicity_st,gap_st,speeding_freq_st,vehicle_mass_st,brakes_st,serv_brake_PE_st,second_brake_st,parking_brake_st,axle_st,warn_lamp_st,door_st,fog_lamp_st,headlamp_st,reverse_lamp_st,belts_st,airbag_st,seat_st,steering_st,wheel_alignment_st,EPS_st,Steering_wheel_st,stop_lamp_st,suspension_st,Telltales_st,wheel_hub_st,wheel_st,tyre_st,cabine_st,chassis_st,noise_st,obt_recog_st,v2v_st,v2i_st,friendly_HM_interaction_st,software_freq_st,biddata_connection_st,digital_user_interface_st,cooperative_driving_st,road_surface_st,road_condition_st,prob_acc_road_st,prob_contruction_st,cab_temperature_st,cab_humidity_st,driving_env_condition_st,weather_st,time_of_day_st] = input_collision_affect(driver_age_st,driver_alcohol_st,driver_alertness_st,driver_vision_st,driver_work_load_st,driver_emotion_st,driver_attitude_st,maintenance_periodicity_st,gap_st,speeding_freq_st,vehicle_mass_st,brakes_st,serv_brake_PE_st,second_brake_st,parking_brake_st,axle_st,warn_lamp_st,door_st,fog_lamp_st,headlamp_st,reverse_lamp_st,belts_st,airbag_st,seat_st,steering_st,wheel_alignment_st,EPS_st,Steering_wheel_st,stop_lamp_st,suspension_st,Telltales_st,wheel_hub_st,wheel_st,tyre_st,cabine_st,chassis_st,noise_st,obt_recog_st,v2v_st,v2i_st,friendly_HM_interaction_st,software_freq_st,biddata_connection_st,digital_user_interface_st,cooperative_driving_st,road_surface_st,road_condition_st,prob_acc_road_st,prob_contruction_st,cab_temperature_st,cab_humidity_st,driving_env_condition_st,weather_st,time_of_day_st,check_if_hit,check_collision)

 rows=54;
    State=zeros(rows,1);
    
    if check_if_hit==1 || check_collision==1
        State(1)=5;
        State(2)=5;
        State(3)=5;
        State(4)=5;
        State(5)=5;
        State(6)=5;
        State(7)=5;
        State(8)=5;
        State(9)=2;
        State(10)=5;
        State(11)=5;
        State(12)=3;
        State(13)=3;
        State(14)=3;
        State(15)=3;
        State(16)=3;
        State(17)=3;
        State(18)=3;
        State(19)=3;
        State(20)=3;
        State(21)=3;
        State(22)=3;
        State(23)=3;
        State(24)=3;
        State(25)=3;
        State(26)=3;
        State(27)=3;
        State(28)=3;
        State(29)=3;
        State(30)=3;
        State(31)=3;
        State(32)=3;
        State(33)=3;
        State(34)=3;
        State(35)=3;
        State(36)=3;
        State(37)=3;
        State(38)=5;
        State(39)=2;
        State(40)=2;
        State(41)=3;
        State(42)=5;
        State(43)=2;
        State(44)=3;
        State(45)=2;
        State(46)=5;
        State(47)=3;
        State(48)=5;
        State(49)=5;
        State(50)=5;
        State(51)=5;
        State(52)=5;
        State(53)=5;
        State(54)=5;
    else
    
        State(1)=driver_age_st;
        State(2)=driver_alcohol_st;
        State(3)=driver_alertness_st;
        State(4)=driver_vision_st;
        State(5)=driver_work_load_st;
        State(6)=driver_emotion_st;
        State(7)=driver_attitude_st;
        State(8)=maintenance_periodicity_st;
        State(9)=gap_st;
        State(10)=speeding_freq_st;
        State(11)=vehicle_mass_st;
        State(12)=brakes_st;
        State(13)=serv_brake_PE_st;
        State(14)=second_brake_st;
        State(15)=parking_brake_st;
        State(16)=axle_st;
        State(17)=warn_lamp_st;
        State(18)=door_st;
        State(19)=fog_lamp_st;
        State(20)=headlamp_st;
        State(21)=reverse_lamp_st;
        State(22)=belts_st;
        State(23)=airbag_st;
        State(24)=seat_st;
        State(25)=steering_st;
        State(26)=wheel_alignment_st;
        State(27)=EPS_st;
        State(28)=Steering_wheel_st;
        State(29)=stop_lamp_st;
        State(30)=suspension_st;
        State(31)=Telltales_st;
        State(32)=wheel_hub_st;
        State(33)=wheel_st;
        State(34)=tyre_st;
        State(35)=cabine_st;
        State(36)=chassis_st;
        State(37)=noise_st;
        State(38)=obt_recog_st;
        State(39)=v2v_st;
        State(40)=v2i_st;
        State(41)=friendly_HM_interaction_st;
        State(42)=software_freq_st;
        State(43)=biddata_connection_st;
        State(44)=digital_user_interface_st;
        State(45)=cooperative_driving_st;
        State(46)=road_surface_st;
        State(47)=road_condition_st;
        State(48)=prob_acc_road_st;
        State(49)=prob_contruction_st;
        State(50)=cab_temperature_st;
        State(51)=cab_humidity_st;
        State(52)=driving_env_condition_st;
        State(53)=weather_st;
        State(54)=time_of_day_st;
    end
    driver_age_st=State(1);
    driver_alcohol_st=State(2);
    driver_alertness_st=State(3);
    driver_vision_st=State(4);
    driver_work_load_st=State(5);
    driver_emotion_st=State(6);
    driver_attitude_st=State(7);
    maintenance_periodicity_st=State(8);
    gap_st=State(9);
    speeding_freq_st=State(10);
    vehicle_mass_st=State(11);
    brakes_st=State(12);
    serv_brake_PE_st=State(13);
    second_brake_st=State(14);
    parking_brake_st=State(15);
    axle_st=State(16);
    warn_lamp_st=State(17);
    door_st=State(18);
    fog_lamp_st=State(19);
    headlamp_st=State(20);
    reverse_lamp_st=State(21);
    belts_st=State(22);
    airbag_st=State(23);
    seat_st=State(24);
    steering_st=State(25);
    wheel_alignment_st=State(26);
    EPS_st=State(27);
    Steering_wheel_st=State(28);
    stop_lamp_st=State(29);
    suspension_st=State(30);
    Telltales_st=State(31);
    wheel_hub_st=State(32);
    wheel_st=State(33);
    tyre_st=State(34);
    cabine_st=State(35);
    chassis_st=State(36);
    noise_st=State(37);
    obt_recog_st=State(38);
    v2v_st=State(39);
    v2i_st=State(40);
    friendly_HM_interaction_st=State(41);
    software_freq_st=State(42);
    biddata_connection_st=State(43);
    digital_user_interface_st=State(44);
    cooperative_driving_st=State(45);
    road_surface_st=State(46);
    road_condition_st=State(47);
    prob_acc_road_st=State(48);
    prob_contruction_st=State(49);
    cab_temperature_st=State(50);
    cab_humidity_st=State(51);
    driving_env_condition_st=State(52);
    weather_st=State(53);
    time_of_day_st=State(54);


end
